simulink model "levelnpc1"  (R2013b)
settings: Solver=ode1  StartTime=0.0  StopTime=15  FixedStep=Ts  RelTol=1e-3
InitFcn:
  | Ts=5e-5
undefined symbols (not defined in the file or in its folder): D1, Delta
libraries: powerlib x34, powerlib_meascontrol x3, simulink x1
settings Model: Creator=LiberT  LastModifiedBy=LiberT
settings DataIOCC: SignalLoggingSaveFormat=ModelDataLogs
settings OptimizationCC: ExpressionDepthLimit=2147483647
settings DebuggingCC: MultiTaskDSMMsg=warning  MultiTaskCondExecSysMsg=none  FcnCallInpInsideContextMsg=EnableAllAsWarning  StateNameClashWarn=warning
settings RTWCC: IncludeERTFirstTime=on

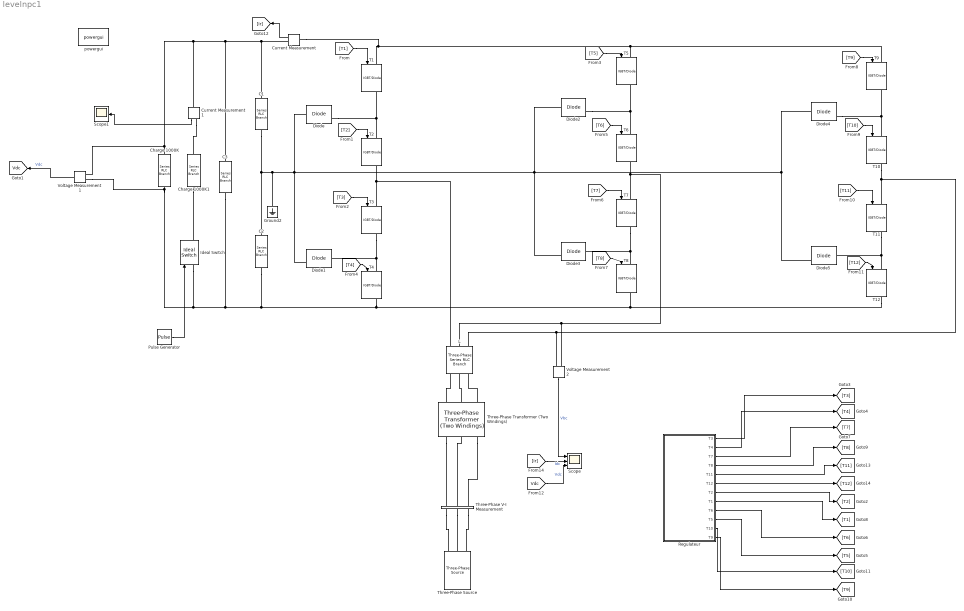
== system levelnpc1 ==
  C1 : powerlib/Elements/Series RLC Branch  LConnTagsString=__new0  RConnTagsString=__new0  BranchType=C  Resistance=1  Inductance=1e-3  SetiL0=off  InitialCurrent=0  Capacitance=1e-9  Setx0=off  InitialVoltage=0  Measurements=None
  C2 : powerlib/Elements/Series RLC Branch  LConnTagsString=__new0  RConnTagsString=__new0  BranchType=C  Resistance=1  Inductance=1e-3  SetiL0=off  InitialCurrent=0  Capacitance=1e-9  Setx0=off  InitialVoltage=0  Measurements=None
  C3 : powerlib/Elements/Series RLC Branch  LConnTagsString=__new0  RConnTagsString=__new0  BranchType=C  Resistance=1  Inductance=1e-3  SetiL0=off  InitialCurrent=0  Capacitance=300e-3  Setx0=off  InitialVoltage=0  Measurements=None
  Charge 1000K : powerlib/Elements/Series RLC Branch  LConnTagsString=__new0  RConnTagsString=__new0  BranchType=Open circuit  Resistance=1000  Inductance=0.0001  SetiL0=off  InitialCurrent=0  Capacitance=0  Setx0=off  InitialVoltage=0  Measurements=None
  Charge 1000K1 : powerlib/Elements/Series RLC Branch  LConnTagsString=__new0  RConnTagsString=__new0  BranchType=RL  Resistance=0.28  Inductance=0.1  SetiL0=off  InitialCurrent=0  Capacitance=0  Setx0=off  InitialVoltage=0  Measurements=None
  Current Measurement : powerlib/Measurements/Current Measurement  PhasorSimulation=off  OutputType=Complex  PSBequivalent=0
  Current Measurement1 : powerlib/Measurements/Current Measurement  PhasorSimulation=off  OutputType=Complex  PSBequivalent=0
  Diode{,1..5} (6 alike) : powerlib/Power Electronics/Diode  Ron=0.001  Lon=0  Vf=0.8  IC=0  UseSnubber=off  Rs=500  Cs=250e-9  Measurements=on
  Ground2 : powerlib/Elements/Ground  LConnTagsString=a
  Ideal Switch : powerlib/Power Electronics/Ideal Switch  Ron=0.001  Lon=0  IC=0  Rs=1e5  Cs=inf  Measurements=on
  L : powerlib/Elements/Three-Phase Series RLC Branch  LConnTagsString=A|B|C  RConnTagsString=A|B|C  BranchType=RL  Resistance=0.1e-3  Inductance=6.4e-3  Capacitance=inf  Measurements=Branch currents
  Pulse Generator : DiscretePulseGenerator  PulseType=Time based  PulseWidth=5  PhaseDelay=8
  Regulateur : Subsystem  mask(DC Voltage Regulator){Vdc_Ref=5000}
      mask prompts: Vdc_Ref "DC voltage setpoint (V):"
  Scope : Scope  NumInputPorts=3
      settings: TickLabels=on  YMin=-7500~-750~4000  YMax=7500~1250~5100
  Scope1 : Scope
      settings: TickLabels=on  YMin=-4000  YMax=4000  SaveName=ScopeData3
  T{1..12} (12 alike) : powerlib/Power Electronics/IGBT//Diode  Ron=1e-3  Rs=1e5  Cs=inf  Measurements=on
  Three-Phase Transformer (Two Windings) : powerlib/Elements/Three-Phase Transformer (Two Windings)  Winding1Connection=Delta (D1)  UNITS=pu  NominalPower=[ 2500e3 , 50 ]  Winding1=[ 18e3 , 0.004 , 0.04 ]  Winding2Connection=Yg  Winding2=[ 2e3 , 0.004 , 0.04 ]  SetSaturation=off  Rm=500  Lm=500  Saturation=[ 0,0 ; 0.0024,1.2 ; 1.0,1.52 ]  Hysteresis=off  DataFile='hysteresis'  SetInitialFlux=off  InitialFluxes=[ 0.8 , -0.8 , 0.7 ]  Measurements=None  MoreParameters=off  BreakLoop=off  DataType=off  TransfoNumber=1
  Three-Phase V-I Measurement : powerlib/Measurements/Three-Phase V-I Measurement  VoltageMeasurement=phase-to-ground  SetLabelV=on  LabelV=Vabc  Vpu=off  VpuLL=off  CurrentMeasurement=yes  SetLabelI=on  LabelI=Iabc  Ipu=off  Pbase=100e6  Vbase=500e3  OutputType=Complex  PhasorSimulation=off  PSBequivalent=0
  Three-Phase Source : powerlib/Electrical Sources/Three-Phase Source  Voltage=18e3  PhaseAngle=0  Frequency=50  InternalConnection=Yg  SpecifyImpedance=off  Resistance=0.8929  Inductance=16.58e-3  ShortCircuitLevel=2500000  BaseVoltage=18e3  XRratio=7  BusType=swing  Pref=0  Qref=0  Qmin=-inf  Qmax=inf
  Voltage Measurement1 : powerlib/Measurements/Voltage Measurement  PhasorSimulation=off  OutputType=Complex  PSBequivalent=0
  Voltage Measurement2 : powerlib/Measurements/Voltage Measurement  PhasorSimulation=off  OutputType=Complex  PSBequivalent=0
  powergui : powerlib/powergui  Priority=1  SimulationMode=Discrete  SolverType=Tustin  SampleTime=Ts  frequency=60  SPID=off  DisableSnubberDevices=off  DisableRonSwitches=off  DisableVfSwitches=off  SwTol=0  Interpol=off  DisplayEquations=off  frequencyindice=50  Pbase=100e6  ErrMax=1e-4  Iterations=50  UnitsV=kV  UnitsW=MW  FunctionMessages=off  echomessages=off  HookPort=off  EnableUseOfTLC=off  x0status=blocks  RestoreLinks=warning  ResistiveCurrentMeasurement=off  Frange=[0:2:500]  Ylog=off  Xlog=on  ShowGrid=off  save=off  variable=ZData  ZoomFFT=off  StartTime=0.0  cycles=1  DisplayStyle=1  fundamental=60  FreqAxis=off  MaxFrequency=1000  frequencyindicesteady=1  RmsSteady=1  display=off  Ts=0  methode=off
  tag scope: Vdc=global
  wires:
  [T8] -> T8/1
  [T7] -> T7/1
  [T6] -> T6/1
  [T5] -> T5/1
  [T9] -> T9/1
  [T10] -> T10/1
  [T11] -> T11/1
  [T12] -> T12/1
  [T4] -> T4/1
  [T3] -> T3/1
  [T2] -> T2/1
  [T1] -> T1/1
  Current Measurement/1 -> [Ir]
  Voltage Measurement2/1 -> Scope/1  "Vbc"
  Regulateur/8(T1) -> [T1]
  Regulateur/7(T2) -> [T2]
  Regulateur/1(T3) -> [T3]
  Regulateur/2(T4) -> [T4]
  Regulateur/10(T5) -> [T5]
  Regulateur/9(T6) -> [T6]
  Regulateur/3(T7) -> [T7]
  Regulateur/4(T8) -> [T8]
  Regulateur/12(T9) -> [T9]
  Regulateur/11(T10) -> [T10]
  Regulateur/5(T11) -> [T11]
  Regulateur/6(T12) -> [T12]
  Voltage Measurement1/1 -> [Vdc]  "Vdc"
  [Ir] -> Scope/2  "Idc"
  [Vdc] -> Scope/3  "Vdc"
  Pulse Generator/1 -> Ideal Switch/1
  Current Measurement1/1 -> Scope1/1
  connections:
  T3/LConn1 -- T2/RConn1 -- L/RConn1
  T3/RConn1 -- T4/LConn1 -- Diode1/LConn1
  T2/LConn1 -- T1/RConn1 -- Diode/RConn1
  Voltage Measurement2/LConn2 -- T7/LConn1 -- T6/RConn1 -- L/RConn2
  Diode3/LConn1 -- T7/RConn1 -- T8/LConn1
  Diode2/RConn1 -- T6/LConn1 -- T5/RConn1
  T10/RConn1 -- T11/LConn1 -- Voltage Measurement2/LConn1 -- L/RConn3
  Diode5/LConn1 -- T11/RConn1 -- T12/LConn1
  Diode4/RConn1 -- T10/LConn1 -- T9/RConn1
  C1/LConn1 -- Current Measurement/RConn1 -- Current Measurement1/LConn1 -- Voltage Measurement1/LConn1 -- Charge 1000K/RConn1 -- C3/LConn1
  Three-Phase V-I Measurement/LConn1 -- Three-Phase Source/RConn1
  Three-Phase V-I Measurement/LConn2 -- Three-Phase Source/RConn2
  Three-Phase V-I Measurement/LConn3 -- Three-Phase Source/RConn3
  Three-Phase Transformer (Two Windings)/LConn2 -- Three-Phase V-I Measurement/RConn2
  Three-Phase Transformer (Two Windings)/LConn3 -- Three-Phase V-I Measurement/RConn3
  Three-Phase Transformer (Two Windings)/LConn1 -- Three-Phase V-I Measurement/RConn1
  Three-Phase Transformer (Two Windings)/RConn1 -- L/LConn1
  Three-Phase Transformer (Two Windings)/RConn2 -- L/LConn2
  Three-Phase Transformer (Two Windings)/RConn3 -- L/LConn3
  T9/LConn1 -- Current Measurement/LConn1 -- T1/LConn1 -- T5/LConn1
  Charge 1000K/LConn1 -- Voltage Measurement1/LConn2 -- Ideal Switch/LConn1 -- C3/RConn1 -- C2/RConn1 -- T12/RConn1 -- T8/RConn1 -- T4/RConn1
  Charge 1000K1/LConn1 -- Ideal Switch/RConn1
  Current Measurement1/RConn1 -- Charge 1000K1/RConn1
  Diode5/RConn1 -- Diode3/RConn1 -- Diode1/RConn1 -- Ground2/LConn1 -- C1/RConn1 -- C2/LConn1 -- Diode/LConn1 -- Diode2/LConn1 -- Diode4/LConn1

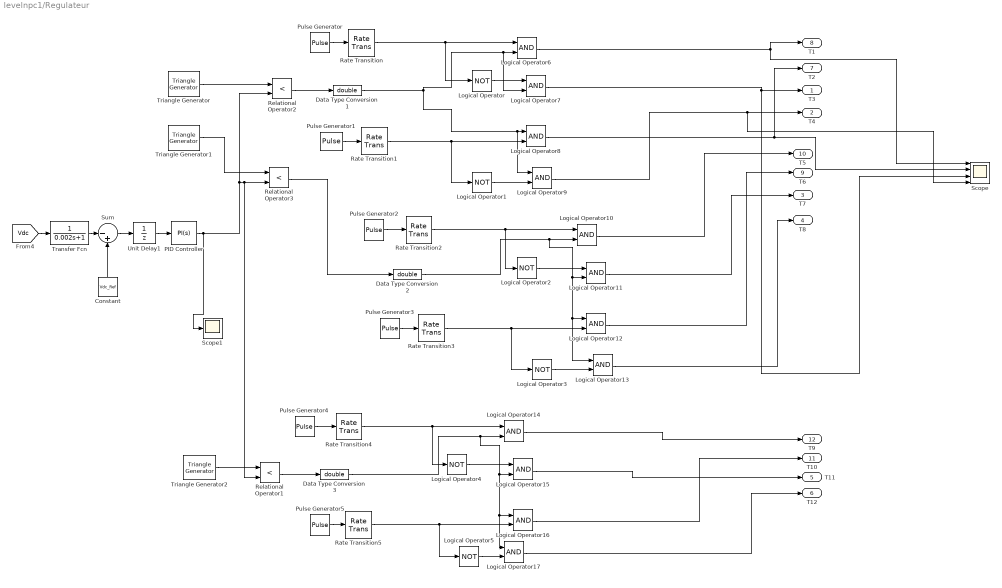
== system levelnpc1/Regulateur ==
  Constant : Constant  Value=Vdc_Ref
  Data Type Conversion1 : DataTypeConversion  OutDataTypeStr=double
  Data Type Conversion2 : DataTypeConversion  OutDataTypeStr=double
  Data Type Conversion3 : DataTypeConversion  OutDataTypeStr=double
  Logical Operator{,1..5} (6 alike) : Logic  Operator=NOT  AllPortsSameDT=off  OutDataTypeStr=boolean
  Logical Operator{6..17} (12 alike) : Logic  AllPortsSameDT=off  OutDataTypeStr=boolean
  PID Controller : simulink/Continuous/PID Controller  Controller=PI  TimeDomain=Continuous-time  SampleTime=1  IntegratorMethod=Forward Euler  FilterMethod=Forward Euler  Form=Parallel  P=0  I=2.8  D=0  N=100  InitialConditionSource=internal  InitialConditionForIntegrator=0  InitialConditionForFilter=0  ExternalReset=none  LimitOutput=on  UpperSaturationLimit=0.95  LowerSaturationLimit=-0.95  LinearizeAsGain=on  AntiWindupMode=clamping  Kb=1  TrackingMode=off  Kt=1  PParamMin=[]  PParamMax=[]  IParamMin=[]  IParamMax=[]  DParamMin=[]  DParamMax=[]  NParamMin=[]  NParamMax=[]  KbParamMin=[]  KbParamMax=[]  KtParamMin=[]  KtParamMax=[]  POutMin=[]  POutMax=[]  IOutMin=[]  IOutMax=[]  DOutMin=[]  DOutMax=[]  NOutMin=[]  NOutMax=[]  KbOutMin=[]  KbOutMax=[]  KtOutMin=[]  KtOutMax=[]  IntegratorOutMin=[]  IntegratorOutMax=[]  FilterOutMin=[]  FilterOutMax=[]  SumOutMin=[]  SumOutMax=[]  SumI1OutMin=[]  SumI1OutMax=[]  SumI2OutMin=[]  SumI2OutMax=[]  SumI3OutMin=[]  SumI3OutMax=[]  SumDOutMin=[]  SumDOutMax=[]  SaturationOutMin=[]  SaturationOutMax=[]  IntegratorContinuousStateAttributes=''  IntegratorStateMustResolveToSignalObject=off  IntegratorRTWStateStorageClass=Auto  FilterContinuousStateAttributes=''  FilterStateMustResolveToSignalObject=off  FilterRTWStateStorageClass=Auto
  Pulse Generator : DiscretePulseGenerator  PulseType=Time based  Period=0.02  PulseWidth=25
  Pulse Generator1 : DiscretePulseGenerator  PulseType=Time based  Period=0.02  PulseWidth=75  PhaseDelay=15e-3
  Pulse Generator2 : DiscretePulseGenerator  PulseType=Time based  Period=0.02  PulseWidth=25  PhaseDelay=0.01
  Pulse Generator3 : DiscretePulseGenerator  PulseType=Time based  Period=0.02  PulseWidth=75  PhaseDelay=25e-3
  Pulse Generator4 : DiscretePulseGenerator  PulseType=Time based  Period=0.02  PulseWidth=25  PhaseDelay=0.02
  Pulse Generator5 : DiscretePulseGenerator  PulseType=Time based  Period=0.02  PulseWidth=75  PhaseDelay=35e-3
  Rate Transition{,1..5} (6 alike) : RateTransition
  Relational Operator1 : RelationalOperator  Operator=<  OutDataTypeStr=boolean
  Relational Operator2 : RelationalOperator  Operator=<  OutDataTypeStr=boolean
  Relational Operator3 : RelationalOperator  Operator=<  OutDataTypeStr=boolean
  Scope : Scope  NumInputPorts=4
      settings: YMin=-0.1~-0.1~-5~-5  YMax=1.1~1.1~5~5  SaveName=ScopeData2
  Scope1 : Scope
  Sum : Sum  Inputs=|-+
  Transfer Fcn : TransferFcn  Denominator=[0.002 1]
  Triangle Generator : powerlib_meascontrol/Pulse & Signal Generators/Triangle Generator  Freq=333  Phase=0  Ts=Ts
  Triangle Generator1 : powerlib_meascontrol/Pulse & Signal Generators/Triangle Generator  Freq=333  Phase=180  Ts=Ts
  Triangle Generator2 : powerlib_meascontrol/Pulse & Signal Generators/Triangle Generator  Freq=333  Phase=360  Ts=Ts
  Unit Delay1 : UnitDelay  SampleTime=-1
  T3 : Outport
  T4 : Outport  Port=2
  T7 : Outport  Port=3
  T8 : Outport  Port=4
  T11 : Outport  Port=5
  T12 : Outport  Port=6
  T2 : Outport  Port=7
  T1 : Outport  Port=8
  T6 : Outport  Port=9
  T5 : Outport  Port=10
  T10 : Outport  Port=11
  T9 : Outport  Port=12
  wires:
  Constant/1 -> Sum/2
  PID Controller/1 -> Scope1/1, Relational Operator2/2, Relational Operator1/2, Relational Operator3/2
  Triangle Generator/1 -> Relational Operator2/1
  Triangle Generator1/1 -> Relational Operator3/1
  Triangle Generator2/1 -> Relational Operator1/1
  Relational Operator2/1 -> Data Type Conversion1/1
  Rate Transition/1 -> Logical Operator6/1, Logical Operator/1
  Rate Transition1/1 -> Logical Operator8/2, Logical Operator1/1
  Data Type Conversion1/1 -> Logical Operator7/2, Logical Operator6/2, Logical Operator9/1, Logical Operator8/1
  Logical Operator6/1 -> T1/1, Scope/1
  Logical Operator/1 -> Logical Operator7/1
  Logical Operator7/1 -> Scope/3, T3/1
  Logical Operator8/1 -> T2/1, Scope/2
  Logical Operator1/1 -> Logical Operator9/2
  Logical Operator9/1 -> Scope/4, T4/1
  Pulse Generator/1 -> Rate Transition/1
  Pulse Generator1/1 -> Rate Transition1/1
  Relational Operator3/1 -> Data Type Conversion2/1
  Rate Transition2/1 -> Logical Operator10/1, Logical Operator2/1
  Rate Transition3/1 -> Logical Operator12/2, Logical Operator3/1
  Data Type Conversion2/1 -> Logical Operator10/2, Logical Operator11/2, Logical Operator13/1, Logical Operator12/1
  Logical Operator2/1 -> Logical Operator11/1
  Logical Operator3/1 -> Logical Operator13/2
  Pulse Generator2/1 -> Rate Transition2/1
  Pulse Generator3/1 -> Rate Transition3/1
  Logical Operator10/1 -> T5/1
  Logical Operator11/1 -> T7/1
  Logical Operator12/1 -> T6/1
  Logical Operator13/1 -> T8/1
  Relational Operator1/1 -> Data Type Conversion3/1
  Rate Transition4/1 -> Logical Operator14/1, Logical Operator4/1
  Rate Transition5/1 -> Logical Operator16/2, Logical Operator5/1
  Data Type Conversion3/1 -> Logical Operator14/2, Logical Operator15/2, Logical Operator17/1, Logical Operator16/1
  Logical Operator14/1 -> T9/1
  Logical Operator4/1 -> Logical Operator15/1
  Logical Operator15/1 -> T11/1
  Logical Operator16/1 -> T10/1
  Logical Operator5/1 -> Logical Operator17/2
  Pulse Generator4/1 -> Rate Transition4/1
  Pulse Generator5/1 -> Rate Transition5/1
  Logical Operator17/1 -> T12/1
  [Vdc] -> Transfer Fcn/1
  Transfer Fcn/1 -> Sum/1
  Sum/1 -> Unit Delay1/1
  Unit Delay1/1 -> PID Controller/1
